simulink library "INT_CoVeh_TrqDesCoord"  (R2016b)
settings: Solver=VariableStepAuto  StartTime=0.0  StopTime=10.0  RelTol=1e-3
settings Model: Creator=Administrator  LastModifiedBy=Administrator

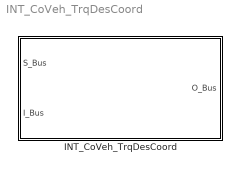
== system INT_CoVeh_TrqDesCoord ==
  INT_CoVeh_TrqDesCoord : Subsystem

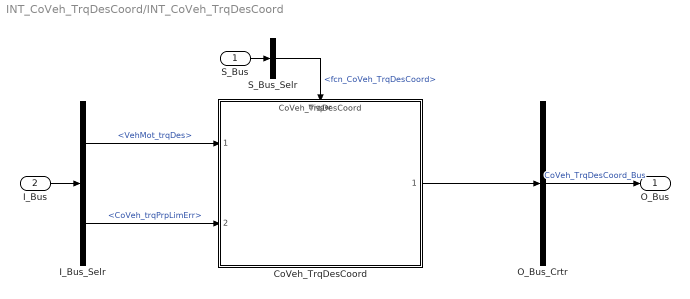
== system INT_CoVeh_TrqDesCoord/INT_CoVeh_TrqDesCoord ==
  S_Bus : Inport
  I_Bus : Inport  Port=2
  CoVeh_TrqDesCoord : ModelReference  ModelNameDialog=CoVeh_TrqDesCoord  SimulationMode=Normal  ModelReferenceVersion=1.2  TriggerPortName=function  TriggerPortTriggerType=function-call  TriggerPortStatesWhenEnabling=held
  I_Bus_Selr : BusSelector  OutputSignals=VehMot_trqDes,CoVeh_trqPrpLimErr
  O_Bus_Crtr : BusCreator  Inputs=1
  S_Bus_Selr : BusSelector  OutputSignals=fcn_CoVeh_TrqDesCoord
  O_Bus : Outport
  wires:
  S_Bus_Selr/1 -> CoVeh_TrqDesCoord/Trigger  "<fcn_CoVeh_TrqDesCoord>"
  S_Bus/1 -> S_Bus_Selr/1
  I_Bus/1 -> I_Bus_Selr/1
  I_Bus_Selr/1 -> CoVeh_TrqDesCoord/1  "<VehMot_trqDes>"
  I_Bus_Selr/2 -> CoVeh_TrqDesCoord/2  "<CoVeh_trqPrpLimErr>"
  O_Bus_Crtr/1 -> O_Bus/1  "CoVeh_TrqDesCoord_Bus"
  CoVeh_TrqDesCoord/1 -> O_Bus_Crtr/1
